simulink model "ContactorMgmt_Harness1"  (R2022b)
settings: configuration reference "BMS_Sw_CodeGenConfig" (kept outside this file)
libraries: SignalEditorBlockLib x1
settings Model: DataDictionary=DD_ContactorMgmt.sldd  Creator=cpatel  LastModifiedBy=cpatel
settings ConfigSetRef: SourceName=BMS_Sw_CodeGenConfig

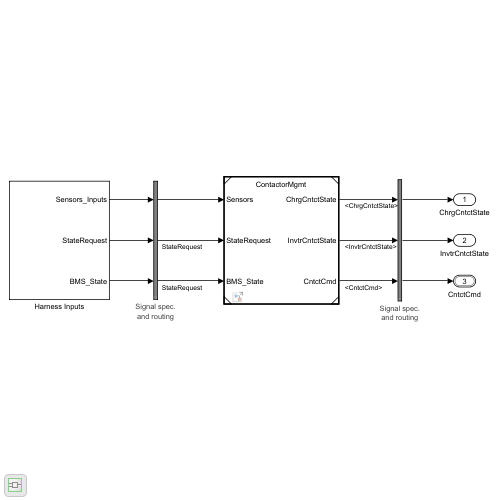
[thumbnail: Simulink's stored preview of the top-level diagram]
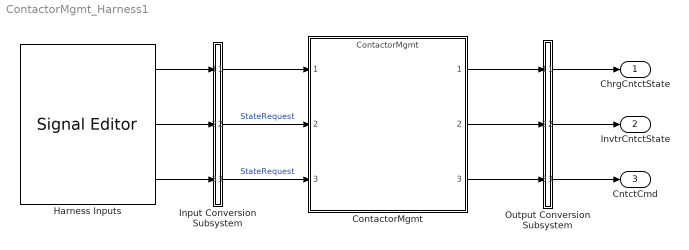
== system ContactorMgmt_Harness1 ==
  ContactorMgmt : ModelReference  ModelNameDialog=ContactorMgmt  SimulationMode=Normal  ModelReferenceVersion=5.0
  Harness Inputs : SignalEditorBlockLib/Signal Editor  FileName=ContactorMgmt_HarnessInputs.mat  ActiveScenario=Charging  ActiveSignal=BMS_State  IsBus=off  OutputBusObjectStr=Bus: BusObject  SampleTime=0.1  Interpolate=off  ZeroCross=off  OutputAfterFinalValue=Holding final value  Unit=inherit  PreserveSignalName=on
  Input Conversion Subsystem : Subsystem  Tag=__SLT_ICS__  Description=|
      | Signal spec.
      | and routing
      settings: AttributesFormatString=%<Description>
  Output Conversion Subsystem : Subsystem  Tag=__SLT_OCS__  Description=|
      | Signal spec.
      | and routing
      settings: AttributesFormatString=%<Description>
  ChrgCntctState : Outport
  InvtrCntctState : Outport  Port=2
  CntctCmd : Outport  Port=3  OutDataTypeStr=Bus: CntctCmd
  wires:
  Harness Inputs/1 -> Input Conversion Subsystem/1(Inport_1)
  Harness Inputs/2 -> Input Conversion Subsystem/2(Inport_2)
  Harness Inputs/3 -> Input Conversion Subsystem/3(Inport_3)
  Output Conversion Subsystem/1(Outport_1) -> ChrgCntctState/1
  Output Conversion Subsystem/2(Outport_2) -> InvtrCntctState/1
  Output Conversion Subsystem/3(Outport_3) -> CntctCmd/1
  Input Conversion Subsystem/1(Outport_1) -> ContactorMgmt/1
  Input Conversion Subsystem/2(Outport_2) -> ContactorMgmt/2  "StateRequest"
  Input Conversion Subsystem/3(Outport_3) -> ContactorMgmt/3  "StateRequest"
  ContactorMgmt/1 -> Output Conversion Subsystem/1(Inport_1)
  ContactorMgmt/2 -> Output Conversion Subsystem/2(Inport_2)
  ContactorMgmt/3 -> Output Conversion Subsystem/3(Inport_3)

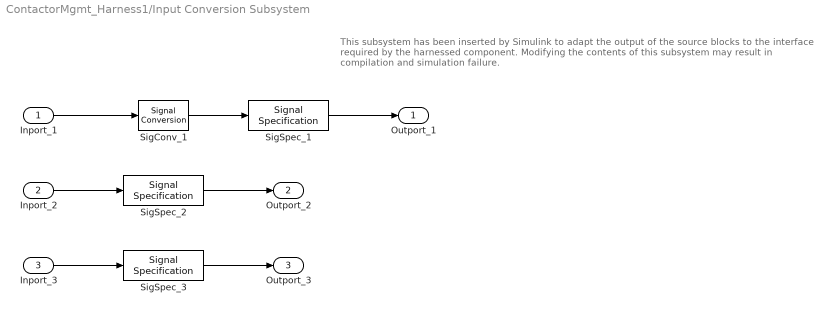
== system ContactorMgmt_Harness1/Input Conversion Subsystem ==
  note: This subsystem has been inserted by Simulink to adapt the output of the source blocks to the interface required by the harnessed component.
      |  Modifying the contents of this subsystem may result in compilation and simulation failure.
  Inport_1 : Inport
  Inport_2 : Inport  Port=2
  Inport_3 : Inport  Port=3
  SigConv_1 : SignalConversion  ConversionOutput=Virtual bus  OverrideOpt=off
  SigSpec_1 : SignalSpecification  OutDataTypeStr=Bus: Sensors  SampleTime=0.1
  SigSpec_2 : SignalSpecification  OutDataTypeStr=Enum: SRE  Dimensions=[1]  SampleTime=0.1
  SigSpec_3 : SignalSpecification  OutDataTypeStr=Enum: BMS_State_Enum  Dimensions=[1]  SampleTime=0.1
  Outport_1 : Outport
  Outport_2 : Outport  Port=2
  Outport_3 : Outport  Port=3
  wires:
  SigSpec_1/1 -> Outport_1/1
  SigConv_1/1 -> SigSpec_1/1
  Inport_1/1 -> SigConv_1/1
  SigSpec_2/1 -> Outport_2/1
  Inport_2/1 -> SigSpec_2/1
  SigSpec_3/1 -> Outport_3/1
  Inport_3/1 -> SigSpec_3/1

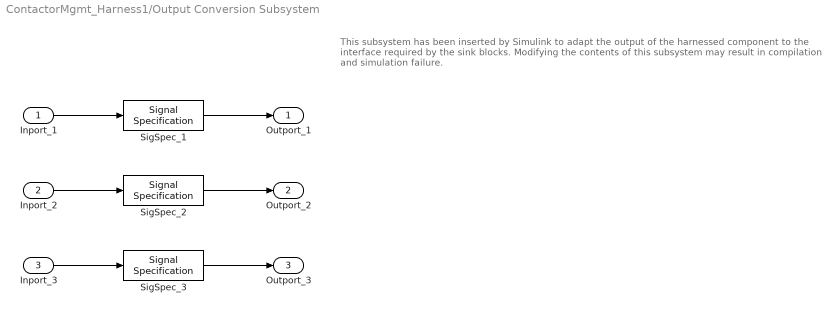
== system ContactorMgmt_Harness1/Output Conversion Subsystem ==
  note: This subsystem has been inserted by Simulink to adapt the output of the harnessed component to the interface required by the sink blocks.
      |  Modifying the contents of this subsystem may result in compilation and simulation failure.
  Inport_1 : Inport
  Inport_2 : Inport  Port=2
  Inport_3 : Inport  Port=3
  SigSpec_1 : SignalSpecification  OutDataTypeStr=Enum: Contact  Dimensions=[1]  SampleTime=0.1
  SigSpec_2 : SignalSpecification  OutDataTypeStr=Enum: Contact  Dimensions=[1]  SampleTime=0.1
  SigSpec_3 : SignalSpecification  OutDataTypeStr=Bus: CntctCmd  Dimensions=[1]  SampleTime=0.1  BusOutputAsStruct=on
  Outport_1 : Outport
  Outport_2 : Outport  Port=2
  Outport_3 : Outport  Port=3
  wires:
  Inport_1/1 -> SigSpec_1/1
  SigSpec_1/1 -> Outport_1/1
  Inport_2/1 -> SigSpec_2/1
  SigSpec_2/1 -> Outport_2/1
  Inport_3/1 -> SigSpec_3/1
  SigSpec_3/1 -> Outport_3/1
